simulink model "Validation_of_model"  (R2024a)
settings: Solver=VariableStepAuto  StartTime=0.0  StopTime=1  MaxStep=1e-5  RelTol=1e-3
values from neighbouring files (symbols this model uses):
  P = 4    [MachineParameters.m]
libraries: PM_BLDC x1, spsCurrentMeasurementLib x1, spsDCVoltageSourceLib x1, simulink x1, spsPermanentMagnetSynchronousMachineLib x1, spsUniversalBridgeLib x1, sps_lib x1
settings Model: PacingRate=0.010000  Creator=Mohamed Draz  LastModifiedBy=Mohamed Draz

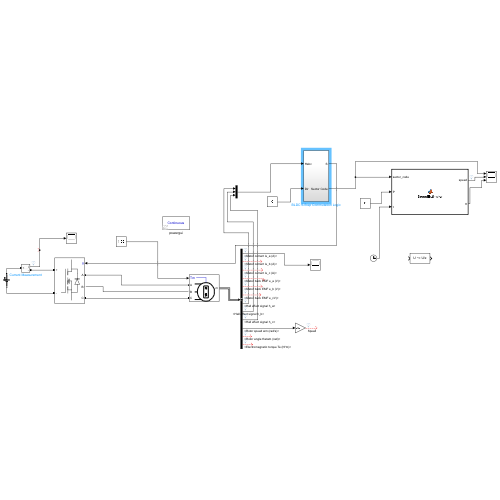
[thumbnail: Simulink's stored preview of the top-level diagram]
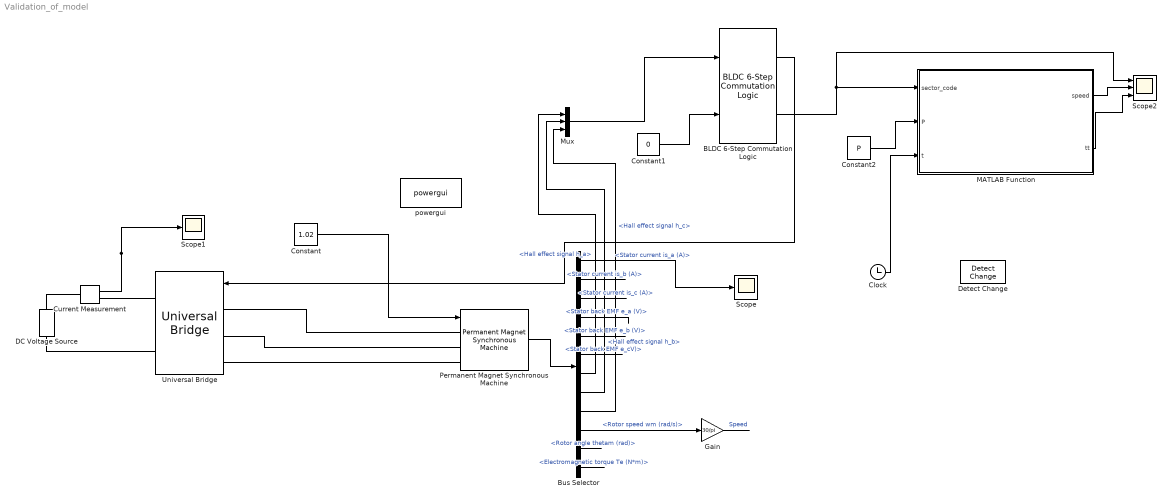
== system Validation_of_model ==
  BLDC 6-Step Commutation Logic : PM_BLDC/BLDC 6-Step Commutation Logic  SystemSampleTime=-1  VariantActivationTime=update diagram  AllowFlexibleInterface=on  Latency=0  AutoFrameSizeCalculation=off
  Bus Selector : BusSelector  OutputSignals=Stator current is_a (A),Stator current is_b (A),Stator current is_c (A),Stator back EMF e_a (V),Stator back EMF e_b (V),Stator back EMF e_cV),Hall effect signal h_a,Hall effect signal h_b,Hall effect signal h_c,Rotor speed wm (rad/s),Rotor angle thetam (rad),Electromagnetic torque Te (N*m)
  Clock : Clock
  Constant : Constant  Value=1.02
  Constant1 : Constant  Value=0
  Constant2 : Constant  Value=P
  Current Measurement : spsCurrentMeasurementLib/Current Measurement  PhasorSimulation=off  OutputType=Complex  PSBequivalent=0
  DC Voltage Source : spsDCVoltageSourceLib/DC Voltage Source  Amplitude=48  Measurements=None
  Detect Change : simulink/Logic and Bit Operations/Detect Change  vinit=0  OutDataTypeStr=boolean
  Gain : Gain  Gain=30/pi
  MATLAB Function : MATLAB Function  TreatAsAtomicUnit=on
  Mux : Mux  Inputs=3
  Permanent Magnet Synchronous Machine : spsPermanentMagnetSynchronousMachineLib/Permanent Magnet Synchronous Machine  NbPhases=3  FluxDistribution=Trapezoidal  RotorType=Round  MechanicalLoad=Torque Tm  PresetModel=No  ShowDetailedParameters=on  MeasurementBus=off  Resistance=0.138  Inductance=0.225e-3  dqInductances=[8.5e-3,8.5e-3]  La=0.000395  MachineConstant=Voltage Constant (V_peak L-L / krpm)  Flux=0.011155  VoltageCst=9.345  TorqueCst=0.089238  Flat=120  Mechanical=[1.7e-5 6.389e-5 4 0]  PolePairs=P  InitialConditions=[0,0, 0,0]  InitialConditions5ph=[0 0 0 0 0 0]  RefAngle=90 degrees behind phase A axis (modified Park)  IterativeDiscreteModel=Trapezoidal non iterative  TsBlock=-1  TsPowergui=0
  Scope : Scope
  Scope1 : Scope
  Scope2 : Scope  NumInputPorts=3
  Universal Bridge : spsUniversalBridgeLib/Universal Bridge  Arms=3  SnubberResistance=1e5  SnubberCapacitance=inf  Device=MOSFET / Diodes  Ron=1e-3  Lon=0  ForwardVoltages="[  0  0  ]"  ForwardVoltage=0  GTOparameters=[ 10e-6 , 20e-6 ]  IGBTparameters=[ 1e-6 , 2e-6 ]  Measurements=None  Measurements_2=None  converterType=Rectifier
  powergui : sps_lib/powergui  Priority=1  SimulationMode=Continuous  SampleTime=50e-6  frequency=60  Iterations=50  frequencyindice=0  Pbase=100e6  ErrMax=1e-4  UnitsV=kV  UnitsW=MW  buscounter=0  FunctionMessages=off  echomessages=off  EnableUseOfTLC=off  CurrentSourceSwitches=off  DisableSnubberDevices=off  DisableRonSwitches=off  DisableVfSwitches=off  DisplayEquations=off  AutomaticDiscreteSolvers=off  SolverType=Tustin/Backward Euler (TBE)  Interpol=off  ExternalGateDelay=off  methode=off  Ts=100  x0status=blocks  SPID=on  SwTol=0  HookPort=off  NonlinearTolerance=1e-4  nMaxIteration=100  ContinueOnMaxIteration=off  RestoreLinks=warning  ResistiveCurrentMeasurement=off  Frange=[0:2:500]  Ylog=off  Xlog=on  ShowGrid=off  save=off  variable=ZData  structure=0  ZoomFFT=off  StartTime=0.0  cycles=1  DisplayStyle=1  fundamental=60  FreqAxis=off  MaxFrequency=1000  frequencyindicesteady=1  RmsSteady=1  display=off
  wires:
  Permanent Magnet Synchronous Machine/1 -> Bus Selector/1
  Mux/1 -> BLDC 6-Step Commutation Logic/1
  Constant1/1 -> BLDC 6-Step Commutation Logic/2
  BLDC 6-Step Commutation Logic/1 -> Universal Bridge/1
  Constant/1 -> Permanent Magnet Synchronous Machine/1
  Bus Selector/1 -> Scope/1  "<Stator current is_a (A)>"
  Bus Selector/2 -> ?  "<Stator current is_b (A)>"
  Bus Selector/3 -> ?  "<Stator current is_c (A)>"
  Bus Selector/6 -> ?  "<Stator back EMF e_cV)>"
  Bus Selector/4 -> ?  "<Stator back EMF e_a (V)>"
  Bus Selector/5 -> ?  "<Stator back EMF e_b (V)>"
  Bus Selector/7 -> Mux/1  "<Hall effect signal h_a>"
  Bus Selector/8 -> Mux/2  "<Hall effect signal h_b>"
  Bus Selector/9 -> Mux/3  "<Hall effect signal h_c>"
  Bus Selector/10 -> Gain/1  "<Rotor speed wm (rad/s)>"
  Bus Selector/11 -> ?  "<Rotor angle thetam (rad)>"
  Bus Selector/12 -> ?  "<Electromagnetic torque Te (N*m)>"
  Gain/1 -> ?  "Speed"
  Current Measurement/1 -> Scope1/1
  BLDC 6-Step Commutation Logic/2 -> Scope2/1, MATLAB Function/1(sector_code)
  MATLAB Function/1(speed) -> Scope2/2
  Constant2/1 -> MATLAB Function/2(P)
  Clock/1 -> MATLAB Function/3(t)
  MATLAB Function/2(tt) -> Scope2/3
  connections:
  DC Voltage Source/LConn1 -- Universal Bridge/RConn2
  Universal Bridge/LConn1 -- Permanent Magnet Synchronous Machine/LConn1
  Universal Bridge/LConn2 -- Permanent Magnet Synchronous Machine/LConn2
  Universal Bridge/LConn3 -- Permanent Magnet Synchronous Machine/LConn3
  DC Voltage Source/RConn1 -- Current Measurement/LConn1
  Current Measurement/RConn1 -- Universal Bridge/RConn1

== matlab function Validation_of_model/MATLAB Function ==
  settings: updateMethod=DISCRETE
  data: sector_code input; speed output; P input; t input; tt output
function [speed, tt]  = SpeedEstimator(sector_code, P, t)

persistent old_sector;
persistent t_old;
persistent Ts;
persistent old_speed;


if isempty(old_sector)
    old_sector = 0;
    t_old = 0;
    old_speed = 0;
    Ts = 0;
    speed = 0;
    tt = Ts;
    return
end

if old_sector ~= sector_code
    Ts = t - t_old;
    old_speed = 1 / (Ts * 6 * P) * 60; % in RPM

    t_old = t;
    old_sector = sector_code;
end

speed = old_speed;
tt = Ts;
